simulink model "GyrosModel"  (R2023b)
settings: Solver=FixedStepDiscrete  StartTime=0.0  StopTime=10  FixedStep=0.001  RelTol=1e-3  EnableMultiTasking=on
values from neighbouring files (symbols this model uses):
  dMaxReadingValue = 300    [main_GyrosModel.m]
  dSamplingTime = 0.1    [main_GyrosModel.m]
settings Model: Creator=peterc  LastModifiedBy=peterc
settings SolverCC: ConcurrentTasks=on  AlgebraicLoopSolver=TrustRegion  PositivePriorityOrder=on  InsertRTBMode=Never (minimum delay)
settings DataIOCC: SaveFormat=Array  SaveState=on  SignalLoggingName=logsOut
settings OptimizationCC: BlockReduction=off  BooleanDataType=off  OptimizeBlockIOStorage=off  BufferReuse=off  ReuseModelBlockBuffer=off  GlobalBufferReuse=off  ExpressionFolding=off  LocalBlockOutputs=off  InitFltsAndDblsToZero=on  OptimizeDataStoreBuffers=off  BusAssignmentInplaceUpdate=off
settings DebuggingCC: SaveWithParameterizedLinksMsg=none  UnderspecifiedInitializationDetection=Classic  MergeDetectMultiDrivingBlocksExec=none  CheckExecutionContextPreStartOutputMsg=on  SignalResolutionControl=TryResolveAllWithWarning  TasksWithSamePriorityMsg=none  UnconnectedInputMsg=warning  UnconnectedOutputMsg=warning  UnconnectedLineMsg=warning  SFUnexpectedBacktrackingDiag=warning  SFNoUnconditionalDefaultTransitionDiag=warning  SFExecutionAtInitializationDiag=none  ArithmeticOperatorsInVariantConditions=warning
settings HardwareCC: ProdBitPerLong=64  ProdLongLongMode=on  ProdHWDeviceType=Intel->x86-64 (Linux 64)
settings ModelReferenceCC: EnableRefExpFcnMdlSchedulingChecks=on  PropagateSignalLabelsOutOfModel=off
settings SFSimCC: SimUseLocalCustomCode=off  SimTargetLang=C++
settings RTWCC: Description=Simulink Real-Time  SystemTargetFile=slrealtime.tlc  TemplateMakefile=slrealtime_default_tmf  RTWUseLocalCustomCode=off  Toolchain=Simulink Real-Time Toolchain  BuildConfiguration=Faster Runs  CodeExecutionProfiling=on  TargetLang=C++  DLArmComputeVersion=19.05
settings CodeAppCC: StateflowObjectComments=on
settings SimulinkRealTimeTargetCC: MATLABClassNameForMDSCustomization=Simulink.SoftwareTarget.GRTCustomization  UseGCCFastMath=on
settings ConfigComp: CovMetricSettings=dw  CovSaveCumulativeToWorkspaceVar=on  CovSaveSingleToWorkspaceVar=on  CovExternalEMLEnable=off  CovSFcnEnable=off

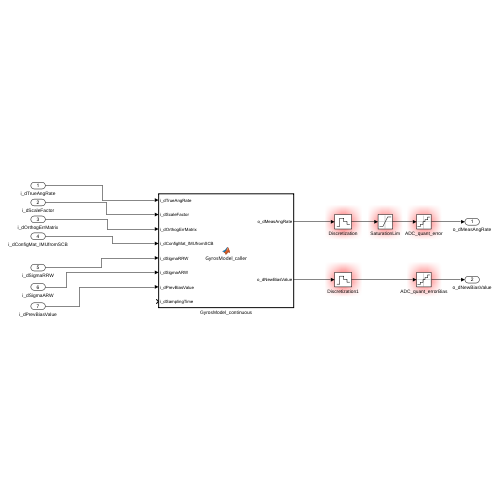
[thumbnail: Simulink's stored preview of the top-level diagram]
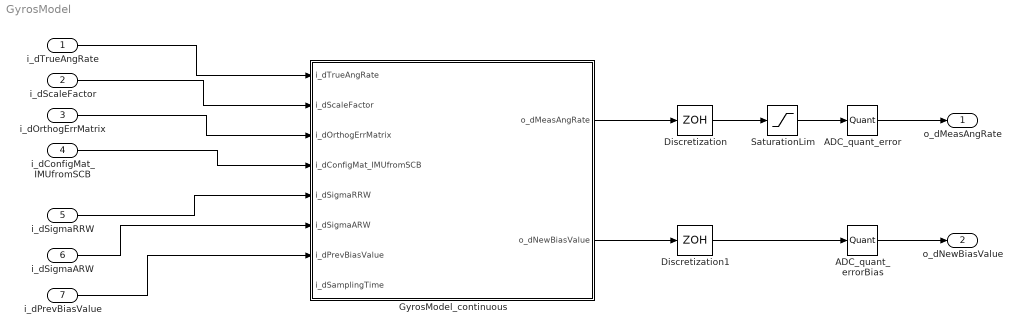
== system GyrosModel ==
  i_dTrueAngRate : Inport  OutDataTypeStr=double  PortDimensions=[3,1]
  i_dScaleFactor : Inport  Port=2  OutDataTypeStr=double  PortDimensions=[3,1]
  i_dOrthogErrMatrix : Inport  Port=3  OutDataTypeStr=double  PortDimensions=[3,3]
  i_dConfigMat_IMUfromSCB : Inport  Port=4  OutDataTypeStr=double  PortDimensions=[3,3]
  i_dSigmaRRW : Inport  Port=5  OutDataTypeStr=double  PortDimensions=[1,1]
  i_dSigmaARW : Inport  Port=6  OutDataTypeStr=double  PortDimensions=[1,1]
  i_dPrevBiasValue : Inport  Port=7  OutDataTypeStr=double  PortDimensions=[3,1]
  ADC_quant_error : Quantizer  QuantizationInterval=QuantizationInterval
  ADC_quant_errorBias : Quantizer  QuantizationInterval=QuantizationInterval
  Discretization : ZeroOrderHold  SampleTime=dSamplingTime
  Discretization1 : ZeroOrderHold  SampleTime=dSamplingTime
  GyrosModel_continuous : MATLAB Function  TreatAsAtomicUnit=on
  SaturationLim : Saturate  UpperLimit=dMaxReadingValue  LowerLimit=-dMaxReadingValue  LinearizeAsGain=off
  o_dMeasAngRate : Outport  OutDataTypeStr=double  PortDimensions=[3,1]
  o_dNewBiasValue : Outport  Port=2  OutDataTypeStr=double  PortDimensions=[3,1]
  wires:
  i_dTrueAngRate/1 -> GyrosModel_continuous/1(i_dTrueAngRate)
  i_dConfigMat_IMUfromSCB/1 -> GyrosModel_continuous/4(i_dConfigMat_IMUfromSCB)
  i_dOrthogErrMatrix/1 -> GyrosModel_continuous/3(i_dOrthogErrMatrix)
  SaturationLim/1 -> ADC_quant_error/1
  i_dScaleFactor/1 -> GyrosModel_continuous/2(i_dScaleFactor)
  ADC_quant_error/1 -> o_dMeasAngRate/1
  Discretization/1 -> SaturationLim/1
  GyrosModel_continuous/2(o_dNewBiasValue) -> Discretization1/1
  ADC_quant_errorBias/1 -> o_dNewBiasValue/1
  Discretization1/1 -> ADC_quant_errorBias/1
  GyrosModel_continuous/1(o_dMeasAngRate) -> Discretization/1
  i_dSigmaARW/1 -> GyrosModel_continuous/6(i_dSigmaARW)
  i_dSigmaRRW/1 -> GyrosModel_continuous/5(i_dSigmaRRW)
  i_dPrevBiasValue/1 -> GyrosModel_continuous/7(i_dPrevBiasValue)

== matlab function GyrosModel/GyrosModel_continuous ==
  data: i_dTrueAngRate input; o_dMeasAngRate output; i_dScaleFactor input; i_dOrthogErrMatrix input; i_dConfigMat_IMUfromSCB input; i_dSigmaRRW input; i_dSigmaARW input; i_dPrevBiasValue input; o_dNewBiasValue output; i_dSamplingTime input
function [o_dMeasAngRate, o_dNewBiasValue] = GyrosModel_caller( i_dTrueAngRate, ...
    i_dScaleFactor          , ...
    i_dOrthogErrMatrix      , ...
    i_dConfigMat_IMUfromSCB , ...
    i_dSigmaRRW             , ...
    i_dSigmaARW             , ...
    i_dPrevBiasValue        ,...
    i_dSamplingTime         ) %#codegen

arguments
    i_dTrueAngRate          (3,1) double    
    i_dScaleFactor          (3,1) double
    i_dOrthogErrMatrix      (3,3) double
    i_dConfigMat_IMUfromSCB (3,3) double
    i_dSigmaRRW             (1,1) double
    i_dSigmaARW             (1,1) double
    i_dPrevBiasValue        (3,1) double
    i_dSamplingTime         (1,1) double
end 

o_dMeasAngRate = zeros(3,1);
o_dNewBiasValue = zeros(3,1);

[o_dMeasAngRate(:), o_dNewBiasValue(:)] = GyrosModel(i_dTrueAngRate, i_dScaleFactor, ...
    i_dOrthogErrMatrix, i_dConfigMat_IMUfromSCB, i_dSigmaRRW, i_dSigmaARW, i_dPrevBiasValue, i_dSamplingTime);%#codegen

end
